simulink model "PMSMmotor_WorkShop"  (R2013b)
settings: Solver=ode45  StartTime=0  StopTime=5  FixedStep=1/fs/4  MaxStep=1/fs  RelTol=1e-7
InitFcn:
  | Motor_parameters_Lsrpm7fw
values from neighbouring files (symbols this model uses):
  fs = 10e3    (= 10000)    [Motor_parameters_Lsrpm7fw.m]
  J = 1*1e-3    (= 0.001)    [Motor_parameters_Lsrpm7fw.m]
  Ki2 = 550    [Motor_parameters_Lsrpm7fw.m]
  Ki3 = 450    [Motor_parameters_Lsrpm7fw.m]
  Kp2 = 6    [Motor_parameters_Lsrpm7fw.m]
  Kp3 = 6    [Motor_parameters_Lsrpm7fw.m]
  Ld = 10e-3    (= 0.01)    [Motor_parameters_Lsrpm7fw.m]
  Lndmpm = 0.412*1    (= 0.412)    [Motor_parameters_Lsrpm7fw.m]
  Lq = 12.8e-3    (= 0.0128)    [Motor_parameters_Lsrpm7fw.m]
  Npp = 8/2    (= 4)    [Motor_parameters_Lsrpm7fw.m]
  Rs = 0.78    [Motor_parameters_Lsrpm7fw.m]
undefined symbols (not defined in the file or in its folder): dfilt, sigbuilder_block
libraries: dsparch4 x3, simulink x1
settings Model: Creator=klu  LastModifiedBy=marcos
settings DataIOCC: SignalLoggingSaveFormat=ModelDataLogs
settings OptimizationCC: BooleanDataType=off  ExpressionDepthLimit=2147483647  InitFltsAndDblsToZero=on
settings DebuggingCC: AlgebraicLoopMsg=none  SaveWithParameterizedLinksMsg=none  SignalResolutionControl=TryResolveAllWithWarning  SolverPrmCheckMsg=none  MultiTaskDSMMsg=warning  MultiTaskCondExecSysMsg=none  FcnCallInpInsideContextMsg=UseLocalSettings  StateNameClashWarn=warning
settings RTWCC: IncludeERTFirstTime=on
settings GRTTargetCC: TargetFcnLib=ansi_tfl_tmw.mat  CombineOutputUpdateFcns=off  GRTInterface=on

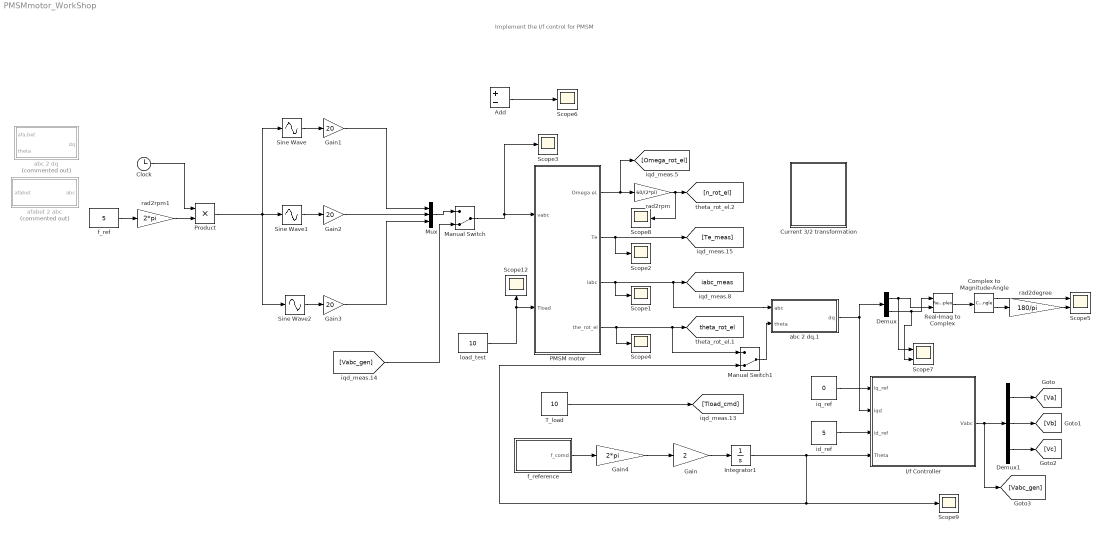
== system PMSMmotor_WorkShop ==
  note: Implement the I/f control for PMSM
  Add : Sum  Inputs=+-
  Clock : Clock
  Complex to Magnitude-Angle : ComplexToMagnitudeAngle
  Current 3/2 transformation : Subsystem
      mask Display:
      | plot([0.1000    0.1357    0.1714    0.2071    0.2429    0.2786    0.3143    0.3500    0.3857    0.4214 0.4571    0.4929    0.5286    0.5643    0.6000]-0.05,0.4+0.6*[0.5000    0.5868    0.6564    0.6950    0.6950    0.6564    0.5868    0.5000    0.4132    0.3436 0.3050    0.3050    0.3436    0.4132    0.5000])
      | 
      | plot([0.1,0.9],[0.1,0.9])
      | 
      | plot([0.5,0.9],0.3*[1 1])
  Demux : Demux  Outputs=2
  Demux1 : Demux  Outputs=3
  Gain : Gain  Gain=2
  Gain1 : Gain  Gain=20
  Gain2 : Gain  Gain=20
  Gain3 : Gain  Gain=20
  Gain4 : Gain  Gain=2*pi
  I/f Controller : Subsystem
  Integrator1 : Integrator  InitialCondition=pi/2
  Manual Switch : ManualSwitch  CurrentSetting=0
  Manual Switch1 : ManualSwitch  CurrentSetting=0
  Mux : Mux  Inputs=3
  PMSM motor : Subsystem
  Product : Product
  Real-Imag to Complex : RealImagToComplex
  Scope{1..4,6,8..9,12} (8 alike) : Scope
      Scope1 settings: TimeRange=0.09507640067911714  YMin=-1.2e-12  YMax=1.2e-12  SaveName=ScopeData22
      Scope12 settings: YMin=0.1  YMax=1.2  SaveName=ScopeData16
      Scope2 settings: TimeRange=2  YMin=5.34264e-13  YMax=5.34264e-13  SaveName=ScopeData4
      Scope3 settings: TimeRange=2  YMin=-50000  YMax=110000  SaveName=ScopeData2
      Scope4 settings: TimeRange=0.09507640067911714  YMin=3  YMax=6.25
      Scope6 settings: TimeRange=2  YMin=-1.75  YMax=1.75  SaveName=ScopeData5
      Scope8 settings: TimeRange=0.09507640067911714  YMin=300  YMax=300  SaveName=ScopeData23
      Scope9 settings: TimeRange=1.4  YMin=1.5  YMax=5.5  SaveName=ScopeData7
  Scope5 : Scope  NumInputPorts=2
      settings: TimeRange=2  YMin=0~-100  YMax=4.25~100  SaveName=ScopeData3
  Scope7 : Scope  NumInputPorts=2
      settings: TimeRange=2  YMin=-4.5~-1.5e-15  YMax=4.5~1.5e-15  SaveName=ScopeData6
  Sine Wave : Sin  TimeSource=Use external signal  Phase=pi/2+0  SampleTime=0
  Sine Wave1 : Sin  TimeSource=Use external signal  Phase=pi/2-pi*2/3  SampleTime=0
  Sine Wave2 : Sin  TimeSource=Use external signal  Phase=pi/2+pi*2/3  SampleTime=0
  T_load : Constant  Value=10
  abc 2 dq : Subsystem  Commented=on
  abc 2 dq.1 : Subsystem
  afabet 2 abc : Subsystem  Commented=on
  f_ref : Constant  Value=5
  f_reference : Subsystem  Tag=STV Subsys  LoadFcn=sigbuilder_block('load');  StartFcn=sigbuilder_block('start');  StopFcn=sigbuilder_block('stop');  ClipboardFcn=sigbuilder_block('clipboard');  mask(Sigbuilder block){}
      mask help: Simulink:masks:SigbuilderBlock_MD
      mask init:
      | if ~strcmp(get_param(bdroot(gcbh),'SimulationStatus'),'stopped') tuvar = sigbuilder_block('maskInit'); end
      settings: CopyFcn=sigbuilder_block('copy');  DeleteFcn=sigbuilder_block('delete');  ModelCloseFcn=sigbuilder_block('modelClose');  PreSaveFcn=sigbuilder_block('preSave');  PauseFcn=sigbuilder_block('pause');  ContinueFcn=sigbuilder_block('continue');  NameChangeFcn=sigbuilder_block('namechange');  OpenFcn=sigbuilder_block('open',[437.25 117.75 550.5 395.25 ]);  CloseFcn=sigbuilder_block('close');
      mask Display: plot(0, 0, 100, 100,[2, 2, 32, 32, 2], [68, 8, 8, 68, 68],[32, 2], [38, 38], [32, 19, 2],[53, 60, 44], [32, 17, 17, 2],[16, 16, 31, 31]);txt = getActiveGroup(gcbh);text(2, 100, txt,'verticalAlignment', 'top');
  id_ref : Constant  Value=5
  iq_ref : Constant  Value=0
  load_test : Constant  Value=10
  rad2degree : Gain  Gain=180/pi
  rad2rpm : Gain  Gain=60/(2*pi)
  rad2rpm1 : Gain  Gain=2*pi
  tag scope: iabc_meas=global, theta_rot_el=global
  wires:
  PMSM motor/2(Te) -> Scope2/1, [Te_meas]
  PMSM motor/1(Omega el.) -> [Omega_rot_el], rad2rpm/1
  PMSM motor/3(iabc) -> abc 2 dq.1/1(abc), [iabc_meas], Scope1/1
  PMSM motor/4(the_rot_el) -> Manual Switch1/1, [theta_rot_el], Scope4/1
  f_reference/1(f_comd) -> Gain4/1
  T_load/1 -> [Tload_cmd]
  rad2rpm/1 -> Scope8/1, [n_rot_el]
  f_ref/1 -> rad2rpm1/1
  Clock/1 -> Product/1
  rad2rpm1/1 -> Product/2
  Product/1 -> Sine Wave/1, Sine Wave1/1, Sine Wave2/1
  Sine Wave/1 -> Gain1/1
  Sine Wave2/1 -> Gain3/1
  abc 2 dq.1/1(dq) -> I/f Controller/2(iqd), Demux/1
  Demux/1 -> Scope7/1, Real-Imag to Complex/2
  Demux/2 -> Scope7/2, Real-Imag to Complex/1
  Real-Imag to Complex/1 -> Complex to Magnitude-Angle/1
  Complex to Magnitude-Angle/1 -> Scope5/1
  Complex to Magnitude-Angle/2 -> rad2degree/1
  rad2degree/1 -> Scope5/2
  Add/1 -> Scope6/1
  load_test/1 -> PMSM motor/2(Tload), Scope12/1
  iq_ref/1 -> I/f Controller/1(iq_ref)
  id_ref/1 -> I/f Controller/3(id_ref)
  I/f Controller/1(Vabc) -> Demux1/1, [Vabc_gen]
  Demux1/1 -> [Va]
  Demux1/2 -> [Vb]
  Demux1/3 -> [Vc]
  Integrator1/1 -> Manual Switch1/2, Scope9/1, I/f Controller/4(Theta)
  Gain4/1 -> Gain/1
  Gain2/1 -> Mux/2
  Gain1/1 -> Mux/1
  Gain/1 -> Integrator1/1
  Mux/1 -> Manual Switch/1
  [Vabc_gen] -> Manual Switch/2
  Manual Switch/1 -> Scope3/1, PMSM motor/1(vabc)
  Gain3/1 -> Mux/3
  Sine Wave1/1 -> Gain2/1
  Manual Switch1/1 -> abc 2 dq.1/2(theta)

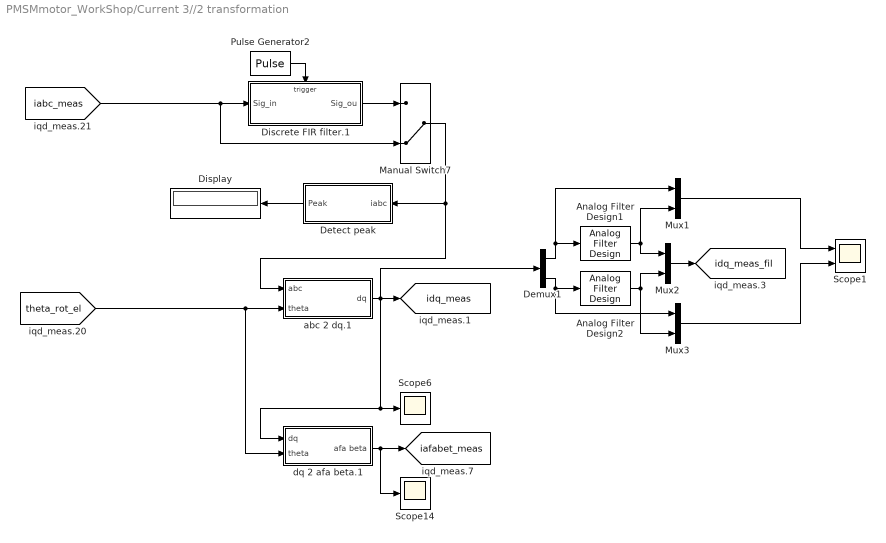
== system PMSMmotor_WorkShop/Current 3//2 transformation ==
  Analog Filter Design1 : dsparch4/Analog Filter Design  method=Butterworth  filttype=Lowpass  N=5  Wlo=2*pi*400  Whi=80  Rp=2  Rs=40
  Analog Filter Design2 : dsparch4/Analog Filter Design  method=Butterworth  filttype=Lowpass  N=5  Wlo=2*pi*400  Whi=80  Rp=2  Rs=40
  Demux1 : Demux  Outputs=2
  Detect peak : Subsystem
  Discrete FIR filter.1 : Subsystem
  Display : Display
  Manual Switch7 : ManualSwitch  CurrentSetting=0
  Mux1 : Mux  Inputs=2
  Mux2 : Mux  Inputs=2
  Mux3 : Mux  Inputs=2
  Pulse Generator2 : DiscretePulseGenerator  PulseType=Time based  Period=1/fs  PulseWidth=50  PhaseDelay=1/fs/4*0
  Scope1 : Scope  NumInputPorts=2
      settings: YMin=-5500~-5  YMax=5500~5  SaveName=ScopeData40
  Scope14 : Scope
      settings: YMin=-5500  YMax=5500  SaveName=ScopeData27
  Scope6 : Scope
      settings: SaveName=ScopeData25
  abc 2 dq.1 : Subsystem
  dq 2 afa beta.1 : Subsystem
  tag scope: iafabet_meas=global, idq_meas=global, idq_meas_fil=global
  wires:
  abc 2 dq.1/1(dq) -> [idq_meas], Demux1/1, Scope6/1, dq 2 afa beta.1/1(dq)
  dq 2 afa beta.1/1(afa beta) -> [iafabet_meas], Scope14/1
  Pulse Generator2/1 -> Discrete FIR filter.1/Trigger
  Manual Switch7/1 -> abc 2 dq.1/1(abc), Detect peak/1(iabc)
  [iabc_meas] -> Discrete FIR filter.1/1(Sig_in), Manual Switch7/2
  Discrete FIR filter.1/1(Sig_ou) -> Manual Switch7/1
  Detect peak/1(Peak) -> Display/1
  [theta_rot_el] -> abc 2 dq.1/2(theta), dq 2 afa beta.1/2(theta)
  Demux1/1 -> Analog Filter Design1/1, Mux1/1
  Demux1/2 -> Analog Filter Design2/1, Mux3/1
  Analog Filter Design1/1 -> Mux2/1, Mux1/2
  Analog Filter Design2/1 -> Mux2/2, Mux3/2
  Mux1/1 -> Scope1/1
  Mux3/1 -> Scope1/2
  Mux2/1 -> [idq_meas_fil]

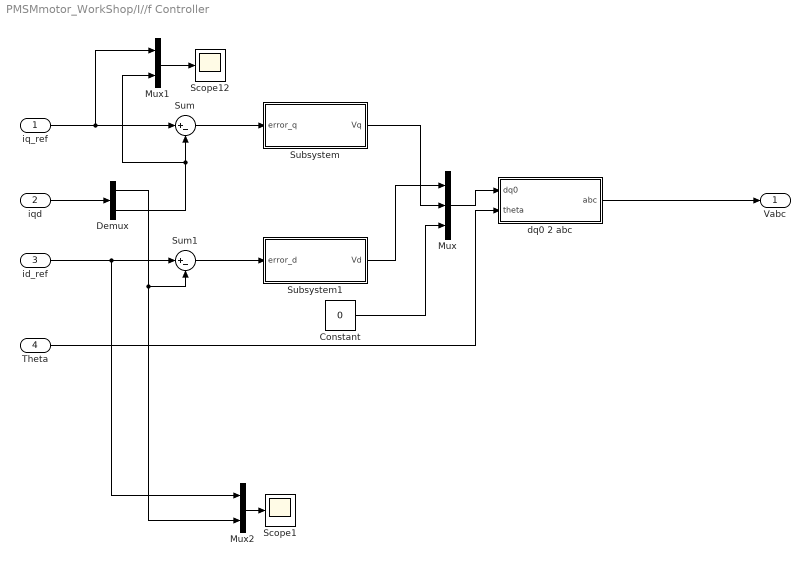
== system PMSMmotor_WorkShop/I//f Controller ==
  iq_ref : Inport
  iqd : Inport  Port=2
  id_ref : Inport  Port=3
  Theta : Inport  Port=4
  Constant : Constant  Value=0
  Demux : Demux  Outputs=2
  Mux : Mux  Inputs=3
  Mux1 : Mux  Inputs=2
  Mux2 : Mux  Inputs=2
  Scope1 : Scope
      settings: YMin=0.1  YMax=1.2  SaveName=ScopeData9
  Scope12 : Scope
      settings: YMin=0.1  YMax=1.2  SaveName=ScopeData8
  Subsystem : Subsystem
  Subsystem1 : Subsystem
  Sum : Sum  Inputs=|+-
  Sum1 : Sum  Inputs=|+-
  dq0 2 abc : Subsystem
  Vabc : Outport
  wires:
  iqd/1 -> Demux/1
  id_ref/1 -> Mux2/1, Sum1/1
  iq_ref/1 -> Mux1/1, Sum/1
  Sum/1 -> Subsystem/1(error_q)
  Sum1/1 -> Subsystem1/1(error_d)
  Mux/1 -> dq0 2 abc/1(dq0)
  Theta/1 -> dq0 2 abc/2(theta)
  dq0 2 abc/1(abc) -> Vabc/1
  Constant/1 -> Mux/3
  Subsystem1/1(Vd) -> Mux/1
  Subsystem/1(Vq) -> Mux/2
  Demux/1 -> Mux2/2, Sum1/2
  Mux1/1 -> Scope12/1
  Demux/2 -> Mux1/2, Sum/2
  Mux2/1 -> Scope1/1

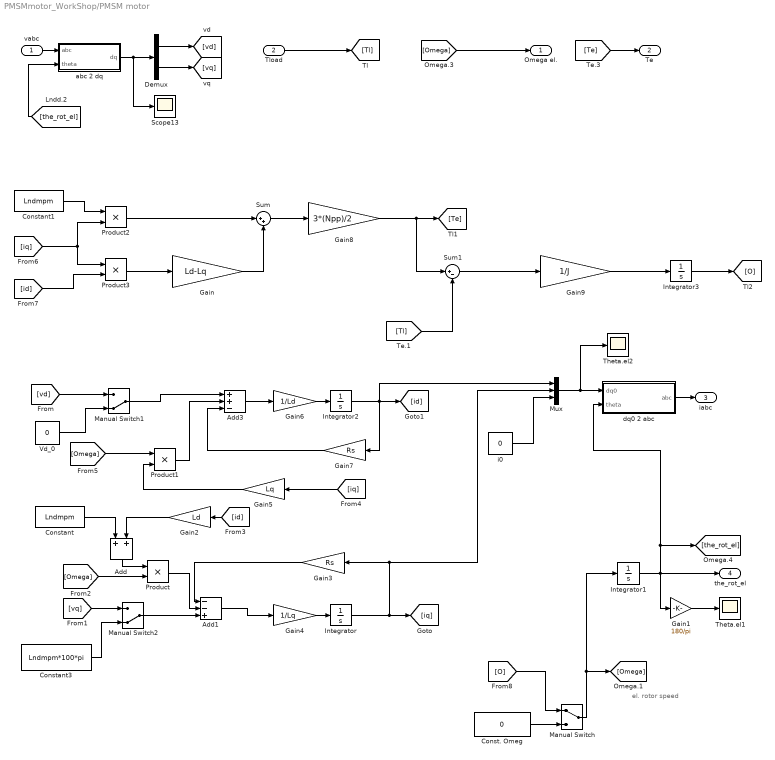
== system PMSMmotor_WorkShop/PMSM motor ==
  note: el. rotor speed
  vabc : Inport
  Tload : Inport  Port=2
  Add : Sum
  Add1 : Sum  Inputs=--+
  Add3 : Sum  Inputs=++-
  Const. Omeg : Constant  Value=0
  Constant : Constant  Value=Lndmpm
  Constant1 : Constant  Value=Lndmpm
  Constant3 : Constant  Value=Lndmpm*100*pi
  Demux : Demux  Outputs=2
  Gain : Gain  Gain=Ld-Lq
  Gain1 : Gain  Gain=180/pi
  Gain2 : Gain  Gain=Ld
  Gain3 : Gain  Gain=Rs
  Gain4 : Gain  Gain=1/Lq
  Gain5 : Gain  Gain=Lq
  Gain6 : Gain  Gain=1/Ld
  Gain7 : Gain  Gain=Rs
  Gain8 : Gain  Gain=3*(Npp)/2
  Gain9 : Gain  Gain=1/J
  Integrator : Integrator
  Integrator1 : Integrator  InitialCondition=pi/2
  Integrator2 : Integrator
  Integrator3 : Integrator
  Manual Switch : ManualSwitch
  Manual Switch1 : ManualSwitch  CurrentSetting=0
  Manual Switch2 : ManualSwitch  CurrentSetting=0
  Mux : Mux  Inputs=3
  Product{,1..3} (4 alike) : Product
  Scope13 : Scope
      settings: YMin=-70  YMax=70  SaveName=ScopeData24
  Sum : Sum  Inputs=|++
  Sum1 : Sum  Inputs=|+-
  Theta.el1 : Scope
      settings: YMin=50  YMax=180
  Theta.el2 : Scope
      settings: YMin=0  YMax=4.25  SaveName=ScopeData10
  Vd_0 : Constant  Value=0
  abc 2 dq : Subsystem
  dq0 2 abc : Subsystem
  i0 : Constant  Value=0
  Omega el. : Outport
  Te : Outport  Port=2
  iabc : Outport  Port=3
  the_rot_el : Outport  Port=4
  wires:
  [Omega] -> Omega el./1
  [Te] -> Te/1
  Tload/1 -> [Tl]
  Demux/2 -> [vq]
  Demux/1 -> [vd]
  dq0 2 abc/1(abc) -> iabc/1
  Integrator1/1 -> Gain1/1, the_rot_el/1, dq0 2 abc/2(theta), [the_rot_el]
  Gain1/1 -> Theta.el1/1
  vabc/1 -> abc 2 dq/1(abc)
  abc 2 dq/1(dq) -> Demux/1, Scope13/1
  [the_rot_el] -> abc 2 dq/2(theta)
  Const. Omeg/1 -> Manual Switch/2
  Manual Switch/1 -> [Omega], Integrator1/1
  Integrator/1 -> Mux/2, Gain3/1, [iq]
  Gain2/1 -> Add/2
  Constant/1 -> Add/1
  [Omega] -> Product/2
  Add/1 -> Product/1
  Gain4/1 -> Integrator/1
  Add1/1 -> Gain4/1
  Product/1 -> Add1/2
  Gain3/1 -> Add1/1
  [id] -> Gain2/1
  [iq] -> Gain5/1
  Gain5/1 -> Product1/2
  [Omega] -> Product1/1
  Product1/1 -> Add3/2
  Add3/1 -> Gain6/1
  Integrator2/1 -> Mux/1, Gain7/1, [id]
  Gain6/1 -> Integrator2/1
  Gain7/1 -> Add3/3
  Mux/1 -> Theta.el2/1, dq0 2 abc/1(dq0)
  i0/1 -> Mux/3
  Constant1/1 -> Product2/1
  [iq] -> Product3/1, Product2/2
  Product2/1 -> Sum/1
  [id] -> Product3/2
  Product3/1 -> Gain/1
  Gain/1 -> Sum/2
  Sum/1 -> Gain8/1
  Gain8/1 -> Sum1/1, [Te]
  [Tl] -> Sum1/2
  Sum1/1 -> Gain9/1
  Gain9/1 -> Integrator3/1
  Integrator3/1 -> [O]
  [O] -> Manual Switch/1
  [vd] -> Manual Switch1/1
  Manual Switch1/1 -> Add3/1
  Vd_0/1 -> Manual Switch1/2
  [vq] -> Manual Switch2/1
  Manual Switch2/1 -> Add1/3
  Constant3/1 -> Manual Switch2/2

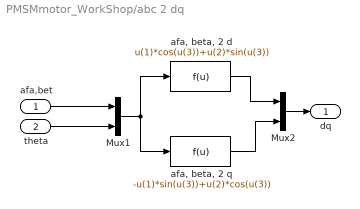
== system PMSMmotor_WorkShop/abc 2 dq ==
  afa,bet : Inport
  theta : Inport  Port=2
  Mux1 : Mux  Inputs=2
  Mux2 : Mux  Inputs=2
  "afa, beta, 2 d" : Fcn  Expr=u(1)*cos(u(3))+u(2)*sin(u(3))
  "afa, beta, 2 q" : Fcn  Expr=-u(1)*sin(u(3))+u(2)*cos(u(3))
  dq : Outport
  wires:
  Mux2/1 -> dq/1
  "afa, beta, 2 q"/1 -> Mux2/2
  "afa, beta, 2 d"/1 -> Mux2/1
  Mux1/1 -> "afa, beta, 2 q"/1, "afa, beta, 2 d"/1
  theta/1 -> Mux1/2
  afa,bet/1 -> Mux1/1

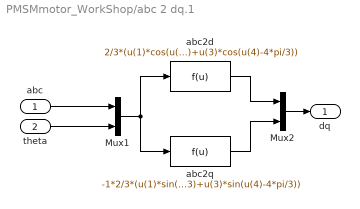
== system PMSMmotor_WorkShop/abc 2 dq.1 ==
  abc : Inport
  theta : Inport  Port=2
  Mux1 : Mux  Inputs=2
  Mux2 : Mux  Inputs=2
  abc2d : Fcn  Expr=2/3*(u(1)*cos(u(4))+u(2)*cos(u(4)-2*pi/3)+u(3)*cos(u(4)-4*pi/3))
  abc2q : Fcn  Expr=-1*2/3*(u(1)*sin(u(4))+u(2)*sin(u(4)-2*pi/3)+u(3)*sin(u(4)-4*pi/3))
  dq : Outport
  wires:
  Mux2/1 -> dq/1
  abc2q/1 -> Mux2/2
  abc2d/1 -> Mux2/1
  Mux1/1 -> abc2q/1, abc2d/1
  theta/1 -> Mux1/2
  abc/1 -> Mux1/1

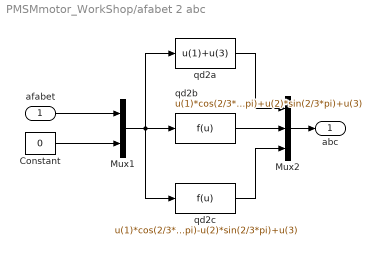
== system PMSMmotor_WorkShop/afabet 2 abc ==
  afabet : Inport
  Constant : Constant  Value=0
  Mux1 : Mux  Inputs=2
  Mux2 : Mux  Inputs=3
  qd2a : Fcn  Expr=u(1)+u(3)
  qd2b : Fcn  Expr=u(1)*cos(2/3*pi)+u(2)*sin(2/3*pi)+u(3)
  qd2c : Fcn  Expr=u(1)*cos(2/3*pi)-u(2)*sin(2/3*pi)+u(3)
  abc : Outport
  wires:
  Constant/1 -> Mux1/2
  qd2c/1 -> Mux2/3
  afabet/1 -> Mux1/1
  Mux1/1 -> qd2c/1, qd2b/1, qd2a/1
  qd2a/1 -> Mux2/1
  qd2b/1 -> Mux2/2
  Mux2/1 -> abc/1

== system PMSMmotor_WorkShop/f_reference ==
  Demux : Demux  Tag=STV Demux  Outputs=1
  FromWs : FromWorkspace  Tag=STV FromWs  VariableName=tuvar  SampleTime=0
      SigBuilderData=|
      | common.afterFinalStr = 'Extrapolate'
      | common.sampleTime = 0
      | dataSet.timeRange = [0 10]
      | dataSet.name = 'Group 1'
      | sbobj.Groups.Name = 'Group 1'
      | sbobj.Groups.Signals.Name = 'f_comd'
      | sbobj.Groups.Signals.XData = [0 1 2 10]
      | sbobj.Groups.Signals.YData = [0 1.005 1 1]
  f_comd : Outport  Tag=STV Outport
  wires:
  FromWs/1 -> Demux/1
  Demux/1 -> f_comd/1

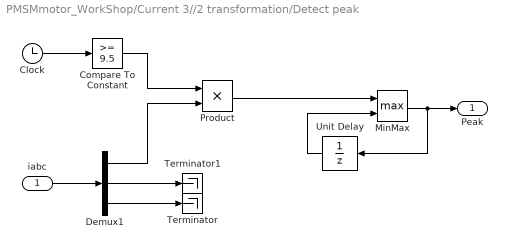
== system PMSMmotor_WorkShop/Current 3//2 transformation/Detect peak ==
  iabc : Inport
  Clock : Clock
  Compare To Constant : simulink/Logic and Bit Operations/Compare To Constant  relop=>=  const=9.5  OutDataTypeStr=uint8  ZeroCross=off
  Demux1 : Demux  Outputs=3
  MinMax : MinMax  Function=max  Inputs=2
  Product : Product  RndMeth=Zero
  Terminator : Terminator
  Terminator1 : Terminator
  Unit Delay : UnitDelay  SampleTime=1/5e3
  Peak : Outport
  wires:
  iabc/1 -> Demux1/1
  Demux1/3 -> Terminator/1
  Demux1/2 -> Terminator1/1
  Clock/1 -> Compare To Constant/1
  Compare To Constant/1 -> Product/1
  Demux1/1 -> Product/2
  MinMax/1 -> Peak/1, Unit Delay/1
  Product/1 -> MinMax/1
  Unit Delay/1 -> MinMax/2

== system PMSMmotor_WorkShop/Current 3//2 transformation/Discrete FIR filter.1 ==
  Sig_in : Inport
  Trigger : TriggerPort
  Filter1 : dsparch4/Digital Filter  Tag=BlockMethodSubSystem  TypePopup=FIR (all zeros)  IIRFiltStruct=Direct form II transposed  AllPoleFiltStruct=Direct form  FIRFiltStruct=Direct form  CoeffSource=Specify via dialog  NumCoeffs=[0.0129982054114534 -0.101337899103369 0.58834244300993 0.58834244300993 -0.101337899103369 0.0129982054114534]  DenCoeffs=[1 0.1]  BiQuadCoeffs=[1 0.3 0.4 1 0.1 0.2]  LatticeCoeffs=[0.2 0.4]  denIgnore=on  FiltPerSampPopup=One filter per frame  IC=0  ICnum=0  ICden=0  roundingMode=Floor  overflowMode=off  ScaleValues=1  scaleValueFracLength=14  stageInFracLength=15  stageOutFracLength=15  FilterSource=Specify via dialog  dfiltObjectName=dfilt.dffir([1 2 1])  InputProcessing=Inherited (this choice will be removed - see release notes)
  Sig_ou : Outport
  wires:
  Sig_in/1 -> Filter1/1
  Filter1/1 -> Sig_ou/1

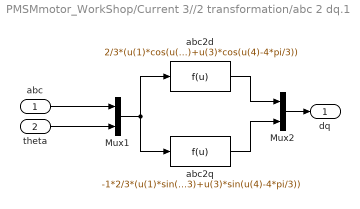
== system PMSMmotor_WorkShop/Current 3//2 transformation/abc 2 dq.1 ==
  abc : Inport
  theta : Inport  Port=2
  Mux1 : Mux  Inputs=2
  Mux2 : Mux  Inputs=2
  abc2d : Fcn  Expr=2/3*(u(1)*cos(u(4))+u(2)*cos(u(4)-2*pi/3)+u(3)*cos(u(4)-4*pi/3))
  abc2q : Fcn  Expr=-1*2/3*(u(1)*sin(u(4))+u(2)*sin(u(4)-2*pi/3)+u(3)*sin(u(4)-4*pi/3))
  dq : Outport
  wires:
  Mux2/1 -> dq/1
  abc2q/1 -> Mux2/2
  abc2d/1 -> Mux2/1
  Mux1/1 -> abc2q/1, abc2d/1
  theta/1 -> Mux1/2
  abc/1 -> Mux1/1

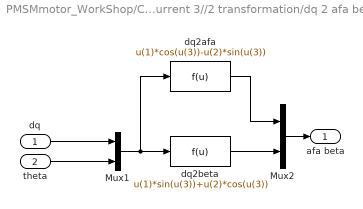
== system PMSMmotor_WorkShop/Current 3//2 transformation/dq 2 afa beta.1 ==
  dq : Inport
  theta : Inport  Port=2
  Mux1 : Mux  Inputs=2
  Mux2 : Mux  Inputs=2
  dq2afa : Fcn  Expr=u(1)*cos(u(3))-u(2)*sin(u(3))
  dq2beta : Fcn  Expr=u(1)*sin(u(3))+u(2)*cos(u(3))
  afa beta : Outport
  wires:
  dq/1 -> Mux1/1
  theta/1 -> Mux1/2
  Mux1/1 -> dq2beta/1, dq2afa/1
  dq2afa/1 -> Mux2/1
  dq2beta/1 -> Mux2/2
  Mux2/1 -> afa beta/1

== system PMSMmotor_WorkShop/I//f Controller/Subsystem ==
  error_q : Inport
  Gain : Gain  Gain=Kp3
  Gain1 : Gain  Gain=Ki3
  Integrator : Integrator
  Sum : Sum  Inputs=|++
  Vq : Outport
  wires:
  error_q/1 -> Gain1/1, Gain/1
  Gain1/1 -> Integrator/1
  Integrator/1 -> Sum/2
  Gain/1 -> Sum/1
  Sum/1 -> Vq/1

== system PMSMmotor_WorkShop/I//f Controller/Subsystem1 ==
  error_d : Inport
  Gain : Gain  Gain=Kp2
  Gain1 : Gain  Gain=Ki2
  Integrator : Integrator
  Sum : Sum  Inputs=|++
  Vd : Outport
  wires:
  error_d/1 -> Gain1/1, Gain/1
  Gain1/1 -> Integrator/1
  Integrator/1 -> Sum/2
  Gain/1 -> Sum/1
  Sum/1 -> Vd/1

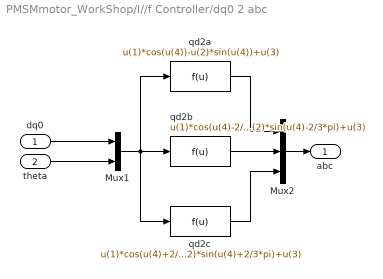
== system PMSMmotor_WorkShop/I//f Controller/dq0 2 abc ==
  dq0 : Inport
  theta : Inport  Port=2
  Mux1 : Mux  Inputs=2
  Mux2 : Mux  Inputs=3
  qd2a : Fcn  Expr=u(1)*cos(u(4))-u(2)*sin(u(4))+u(3)
  qd2b : Fcn  Expr=u(1)*cos(u(4)-2/3*pi)-u(2)*sin(u(4)-2/3*pi)+u(3)
  qd2c : Fcn  Expr=u(1)*cos(u(4)+2/3*pi)-u(2)*sin(u(4)+2/3*pi)+u(3)
  abc : Outport
  wires:
  Mux2/1 -> abc/1
  qd2b/1 -> Mux2/2
  qd2a/1 -> Mux2/1
  Mux1/1 -> qd2b/1, qd2c/1, qd2a/1
  theta/1 -> Mux1/2
  dq0/1 -> Mux1/1
  qd2c/1 -> Mux2/3

== system PMSMmotor_WorkShop/PMSM motor/abc 2 dq ==
  abc : Inport
  theta : Inport  Port=2
  Mux1 : Mux  Inputs=2
  Mux2 : Mux  Inputs=2
  abc2d : Fcn  Expr=-1*2/3*(u(1)*sin(u(4))+u(2)*sin(u(4)-2*pi/3)+u(3)*sin(u(4)-4*pi/3))
  abc2q : Fcn  Expr=2/3*(u(1)*cos(u(4))+u(2)*cos(u(4)-2*pi/3)+u(3)*cos(u(4)-4*pi/3))
  dq : Outport
  wires:
  Mux2/1 -> dq/1
  abc2d/1 -> Mux2/2
  abc2q/1 -> Mux2/1
  Mux1/1 -> abc2d/1, abc2q/1
  theta/1 -> Mux1/2
  abc/1 -> Mux1/1

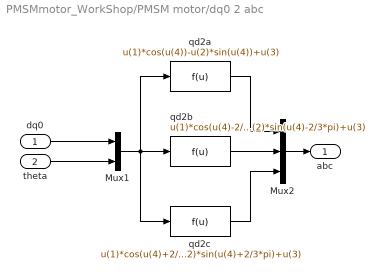
== system PMSMmotor_WorkShop/PMSM motor/dq0 2 abc ==
  dq0 : Inport
  theta : Inport  Port=2
  Mux1 : Mux  Inputs=2
  Mux2 : Mux  Inputs=3
  qd2a : Fcn  Expr=u(1)*cos(u(4))-u(2)*sin(u(4))+u(3)
  qd2b : Fcn  Expr=u(1)*cos(u(4)-2/3*pi)-u(2)*sin(u(4)-2/3*pi)+u(3)
  qd2c : Fcn  Expr=u(1)*cos(u(4)+2/3*pi)-u(2)*sin(u(4)+2/3*pi)+u(3)
  abc : Outport
  wires:
  Mux2/1 -> abc/1
  qd2b/1 -> Mux2/2
  qd2a/1 -> Mux2/1
  Mux1/1 -> qd2b/1, qd2c/1, qd2a/1
  theta/1 -> Mux1/2
  dq0/1 -> Mux1/1
  qd2c/1 -> Mux2/3
